simulink model "EV_ELECTRIC_MOTOR"  (R2023b)
settings: Solver=VariableStepAuto  StartTime=0.0  StopTime=10.0  RelTol=1e-3
settings Model: Creator=HP5CD  LastModifiedBy=HP5CD

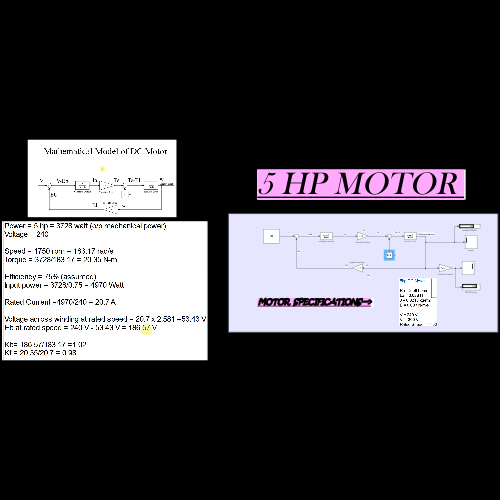
[thumbnail: Simulink's stored preview of the top-level diagram]
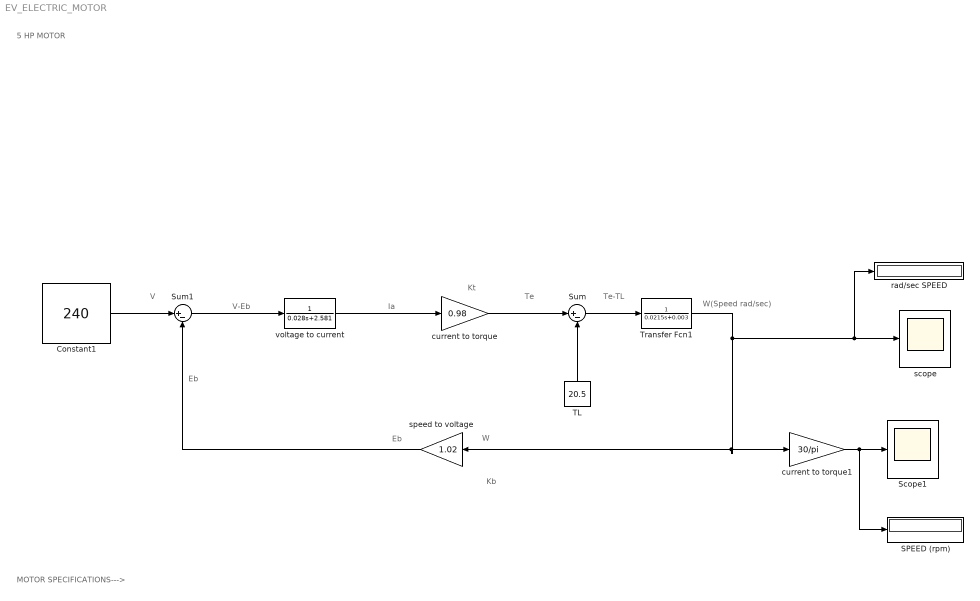
== system EV_ELECTRIC_MOTOR ==
  note: 5 HP MOTOR
  note: Kb
  note: Kt
  note: MOTOR SPECIFICATIONS--->
  note: Eb
  note: W
  note: W(Speed rad/sec)
  note: V
  note: Eb
  note: V-Eb
  note: Ia
  note: Te
  note: Te-TL
  " TL" : Constant  Value=20.5
  Constant1 : Constant  Value=240
  SPEED (rpm) : Display
  Scope1 : Scope
  Sum : Sum  Inputs=|+-
  Sum1 : Sum  Inputs=|+-
  Transfer Fcn1 : TransferFcn  Denominator=[0.0215 0.003]
  current to torque : Gain  Gain=0.98
  current to torque1 : Gain  Gain=30/pi
  rad/sec SPEED : Display
  scope : Scope
  speed to voltage : Gain  Gain=1.02
  voltage to current : TransferFcn  Denominator=[0.028 2.581]
  wires:
  " TL"/1 -> Sum/2
  Sum1/1 -> voltage to current/1
  voltage to current/1 -> current to torque/1
  current to torque/1 -> Sum/1
  Sum/1 -> Transfer Fcn1/1
  Transfer Fcn1/1 -> rad/sec SPEED/1, scope/1, current to torque1/1, speed to voltage/1
  speed to voltage/1 -> Sum1/2
  Constant1/1 -> Sum1/1
  current to torque1/1 -> SPEED (rpm)/1, Scope1/1
